simulink model "sl_quadrotor"  (R2020a)
settings: Solver=VariableStepAuto  StartTime=0.0  StopTime=10.0  RelTol=1e-3
InitFcn:
  | % load parameters of the default quadrotor
  | disp('Quadrotor parameters loaded by PreLoadFcn')
  | mdl_quad
undefined symbols (not defined in the file): dot_x, dot_y, dot_z, Omegax, Omegay, Omegaz, pitch, quadrotor, roll, X, Y, yaw, Z
settings Model: Creator=sw  LastModifiedBy=sw

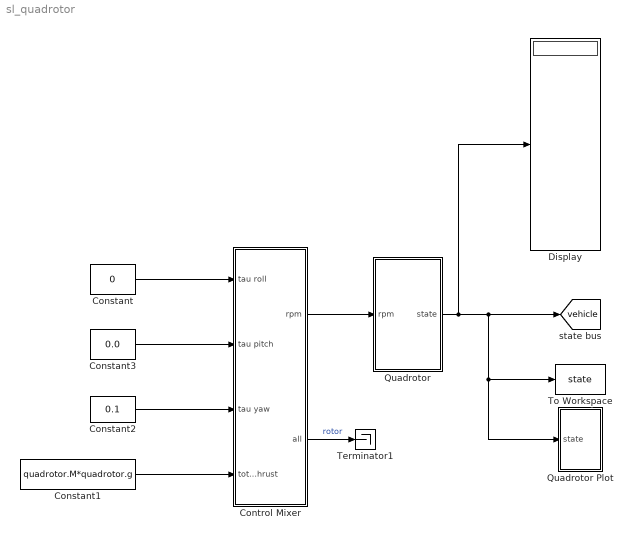
== system sl_quadrotor ==
  Constant : Constant  Value=0
  Constant1 : Constant  Value=quadrotor.M*quadrotor.g
  Constant2 : Constant  Value=0.1
  Constant3 : Constant  Value=0.0
  Control Mixer : Subsystem  mask{quad=quadrotor, maxrot=1000, minrot=5}
      mask prompts: quad "Quadrotor parameters"; maxrot "Maxmun rotor speed(rad/s)"; minrot "Minimun rotor speed(rad/s)"
      mask Display:
      | port_label('output',1,'rpm','texmode','on');
      | port_label('output',2,'\tau_a','texmode','on');
      | port_label('input',1,'\tau_x','texmode','on');
      | port_label('input',2,'\tau_y','texmode','on');
      | port_label('input',3,'\tau_z','texmode','on');
      | port_label('input',4,'T','texmode','on');
  Display : Display
  Quadrotor : Subsystem  mask{quad=quadrotor, x0=[1 1 -1], n0=[0 0 0], groundflag=on}
      mask prompts: quad "Quadrotor params"; x0 "Initial position"; n0 "Initial Ang.(Y,P,R) rad"; groundflag "Ground"
      mask Display:
      | port_label('input',1,'rpm','texmode','on');
      | port_label('output',1,'state','texmode','on');
  Quadrotor Plot : Subsystem  mask{quad=quadrotor, xydim=2, zdim=3, plot=1, enable=1}
      mask prompts: quad "Model"; xydim "xy-axes dimension"; zdim "z-axis dimension"; plot "figure handle"; enable "enable show figure"
  Terminator1 : Terminator
  To Workspace : ToWorkspace  VariableName=state  SampleTime=-1
  tag scope: vehicle=global
  wires:
  Control Mixer/1(rpm) -> Quadrotor/1(rpm)
  Quadrotor/1(state) -> Quadrotor Plot/1(state), To Workspace/1, [vehicle], Display/1
  Constant/1 -> Control Mixer/1(tau roll)
  Constant1/1 -> Control Mixer/4(total thrust)
  Control Mixer/2(all) -> Terminator1/1  "rotor"
  Constant2/1 -> Control Mixer/3(tau yaw)
  Constant3/1 -> Control Mixer/2(tau pitch)

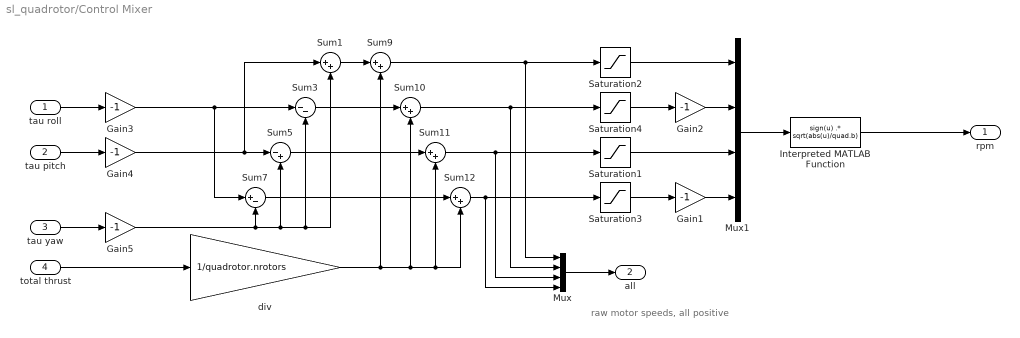
== system sl_quadrotor/Control Mixer ==
  note: raw motor speeds, all positive
  tau roll : Inport
  tau pitch : Inport  Port=2
  tau yaw : Inport  Port=3
  total thrust : Inport  Port=4
  Gain{1..5} (5 alike) : Gain  Gain=-1
  Interpreted MATLAB Function : MATLABFcn  MATLABFcn=sign(u) .* sqrt(abs(u)/quad.b)
  Mux : Mux
  Mux1 : Mux
  Saturation{1..4} (4 alike) : Saturate  UpperLimit=maxrot  LowerLimit=minrot
  Sum{1,9..12} (5 alike) : Sum  Inputs=|++  InputSameDT=on  SaturateOnIntegerOverflow=on  OutDataTypeStr=Inherit: Same as first input
  Sum3 : Sum  Inputs=|--  InputSameDT=on  SaturateOnIntegerOverflow=on  OutDataTypeStr=Inherit: Same as first input
  Sum5 : Sum  Inputs=|-+  InputSameDT=on  SaturateOnIntegerOverflow=on  OutDataTypeStr=Inherit: Same as first input
  Sum7 : Sum  Inputs=|+-  InputSameDT=on  SaturateOnIntegerOverflow=on  OutDataTypeStr=Inherit: Same as first input
  div : Gain  Gain=1/quadrotor.nrotors
  rpm : Outport
  all : Outport  Port=2  VectorParamsAs1DForOutWhenUnconnected=off
  wires:
  Sum9/1 -> Saturation2/1, Mux/1
  Mux/1 -> all/1
  Gain1/1 -> Mux1/4
  Sum12/1 -> Mux/4, Saturation3/1
  Mux1/1 -> Interpreted MATLAB Function/1
  Sum3/1 -> Sum10/1
  Sum1/1 -> Sum9/1
  Sum5/1 -> Sum11/1
  Sum11/1 -> Mux/3, Saturation1/1
  Sum7/1 -> Sum12/1
  Sum10/1 -> Mux/2, Saturation4/1
  Saturation1/1 -> Mux1/3
  Saturation3/1 -> Gain1/1
  Saturation4/1 -> Gain2/1
  div/1 -> Sum10/2, Sum11/2, Sum12/2, Sum9/2
  Saturation2/1 -> Mux1/1
  Gain2/1 -> Mux1/2
  Interpreted MATLAB Function/1 -> rpm/1
  total thrust/1 -> div/1
  tau roll/1 -> Gain3/1
  Gain3/1 -> Sum7/1, Sum3/1
  tau pitch/1 -> Gain4/1
  Gain4/1 -> Sum1/1, Sum5/1
  tau yaw/1 -> Gain5/1
  Gain5/1 -> Sum1/2, Sum3/2, Sum5/2, Sum7/2

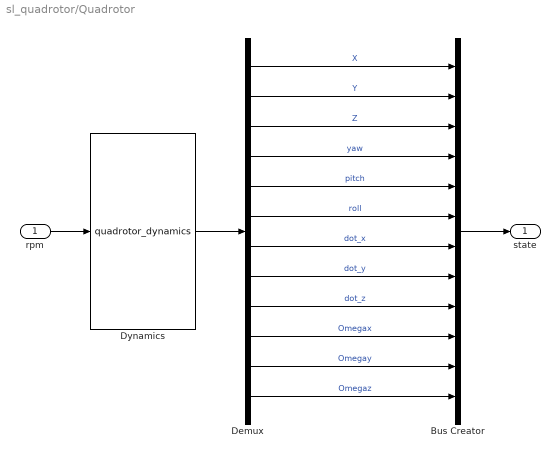
== system sl_quadrotor/Quadrotor ==
  rpm : Inport
  Bus Creator : BusCreator  Inputs=X,Y,Z,yaw,pitch,roll,dot_x,dot_y,dot_z,Omegax,Omegay,Omegaz
  Demux : Demux  Outputs=12
      settings: DisplayOption=none
  Dynamics : S-Function  FunctionName=quadrotor_dynamics  Parameters=quad, x0, n0, groundflag  SFunctionDeploymentMode=off  EnableBusSupport=off
  state : Outport
  wires:
  rpm/1 -> Dynamics/1
  Dynamics/1 -> Demux/1
  Demux/1 -> Bus Creator/1  "X"
  Demux/2 -> Bus Creator/2  "Y"
  Demux/3 -> Bus Creator/3  "Z"
  Demux/4 -> Bus Creator/4  "yaw"
  Demux/5 -> Bus Creator/5  "pitch"
  Demux/6 -> Bus Creator/6  "roll"
  Demux/7 -> Bus Creator/7  "dot_x"
  Demux/8 -> Bus Creator/8  "dot_y"
  Demux/9 -> Bus Creator/9  "dot_z"
  Demux/10 -> Bus Creator/10  "Omegax"
  Demux/12 -> Bus Creator/12  "Omegaz"
  Bus Creator/1 -> state/1
  Demux/11 -> Bus Creator/11  "Omegay"

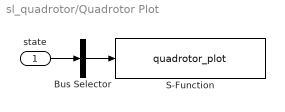
== system sl_quadrotor/Quadrotor Plot ==
  state : Inport
  Bus Selector : BusSelector  OutputSignals=X,Y,Z,yaw,pitch,roll  OutputAsBus=on
  S-Function : S-Function  FunctionName=quadrotor_plot  Parameters=[xydim, zdim], plot, enable,quad  SFunctionDeploymentMode=off  EnableBusSupport=off
  wires:
  Bus Selector/1 -> S-Function/1
  state/1 -> Bus Selector/1
